simulink model "Geometric_Controller"  (R2021a)
settings: Solver=FixedStepAuto  StartTime=0.0  StopTime=40  FixedStep=0.001  RelTol=1e-3
values from neighbouring files (symbols this model uses):
  g = 9.81    [init.m]
  I = 0.025*eye(3)    [init.m]
  m = 1.5    [init.m]
  omega_0 = [0 0 0]    [init.m]
  p_0 = [0 0 0]    [init.m]
  R_0 = eye(3)    [init.m]
  V_0 = [0 0 0]    [init.m]
libraries: vrlib x2, sharedtransform x1
settings Model: Creator=RyllM  LastModifiedBy=RyllM
settings SolverCC: AlgebraicLoopSolver=TrustRegion
settings DataIOCC: ReturnWorkspaceOutputs=off
settings DebuggingCC: SFMachineParentedDataDiag=warning  ArithmeticOperatorsInVariantConditions=warning
settings SFSimCC: SimUseLocalCustomCode=off  CustomCodeUndefinedFunction=UseInterfaceOnly
settings RTWCC: RTWUseLocalCustomCode=off
settings CodeAppCC: StateflowObjectComments=on

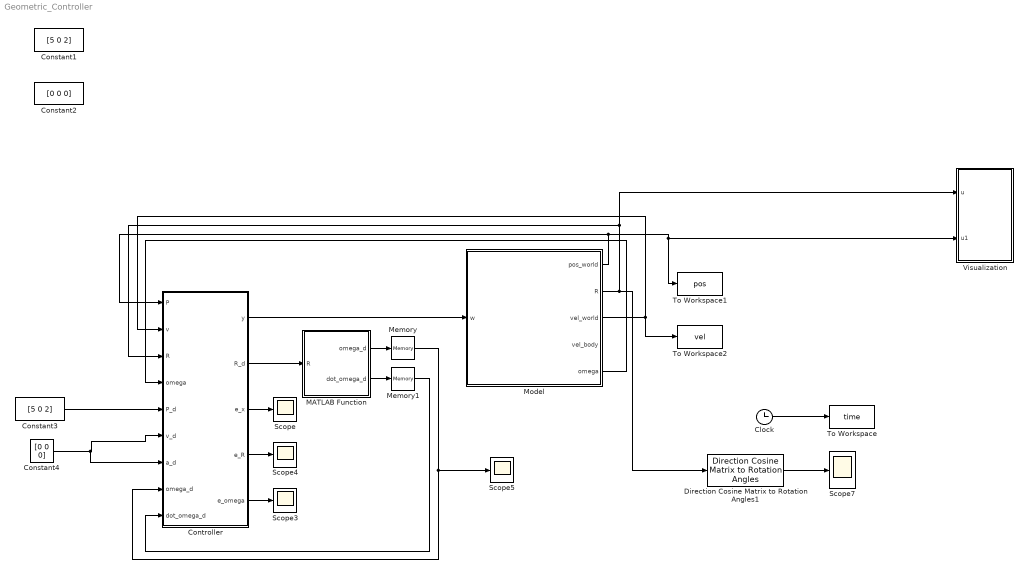
== system Geometric_Controller ==
  Clock : Clock
  Constant1 : Constant  Value=[5 0 2]
  Constant2 : Constant  Value=[0 0 0]
  Constant3 : Constant  Value=[5 0 2]
  Constant4 : Constant  Value=[0 0 0]
  Controller : MATLAB Function  TreatAsAtomicUnit=on
  Direction Cosine Matrix to Rotation Angles1 : sharedtransform/Direction Cosine Matrix to Rotation Angles  rotationOrder=ZYX  aMode=aMode  action=None  tolerance=eps(2)
      settings: SourceProductBaseCode=AE,PW,DR,MT,UV,VE
  MATLAB Function : MATLAB Function  TreatAsAtomicUnit=on
  Memory : Memory  InitialCondition=zeros(3,1)  InheritSampleTime=on
  Memory1 : Memory  InitialCondition=zeros(3,1)  InheritSampleTime=on
  Model : Subsystem
  Scope{,3..5,7} (5 alike) : Scope
  To Workspace : ToWorkspace  VariableName=time  SampleTime=-1
  To Workspace1 : ToWorkspace  VariableName=pos  SampleTime=-1
  To Workspace2 : ToWorkspace  VariableName=vel  SampleTime=-1
  Visualization : Subsystem
  wires:
  Model/1(pos_world) -> Controller/1(P), Visualization/2(u1), To Workspace1/1
  Model/5(omega) -> Controller/4(omega)
  Clock/1 -> To Workspace/1
  Model/3(vel_world) -> Controller/2(v), To Workspace2/1
  Constant4/1 -> Controller/7(a_d), Controller/6(v_d)
  Controller/1(y) -> Model/1(w)
  Controller/3(e_x) -> Scope/1
  Controller/2(R_d) -> MATLAB Function/1(R)
  MATLAB Function/1(omega_d) -> Memory/1
  Memory/1 -> Scope5/1, Controller/8(omega_d)
  Controller/4(e_R) -> Scope4/1
  MATLAB Function/2(dot_omega_d) -> Memory1/1
  Model/2(R) -> Direction Cosine Matrix to Rotation Angles1/1, Visualization/1(u), Controller/3(R)
  Direction Cosine Matrix to Rotation Angles1/1 -> Scope7/1
  Memory1/1 -> Controller/9(dot_omega_d)
  Controller/5(e_omega) -> Scope3/1
  Constant3/1 -> Controller/5(P_d)

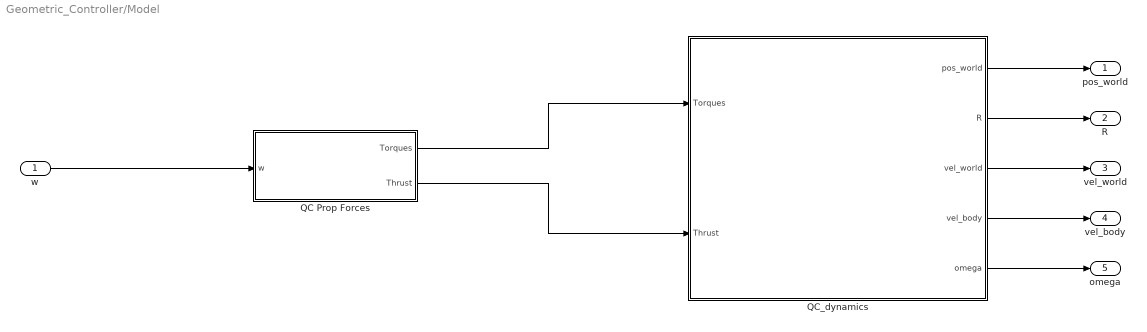
== system Geometric_Controller/Model ==
  w : Inport
  QC Prop Forces : MATLAB Function  TreatAsAtomicUnit=on
  QC_dynamics : Subsystem
  pos_world : Outport
  R : Outport  Port=2
  vel_world : Outport  Port=3
  vel_body : Outport  Port=4
  omega : Outport  Port=5
  wires:
  QC Prop Forces/1(Torques) -> QC_dynamics/1(Torques)
  QC Prop Forces/2(Thrust) -> QC_dynamics/2(Thrust)
  QC_dynamics/1(pos_world) -> pos_world/1
  QC_dynamics/2(R) -> R/1
  QC_dynamics/3(vel_world) -> vel_world/1
  QC_dynamics/4(vel_body) -> vel_body/1
  QC_dynamics/5(omega) -> omega/1
  w/1 -> QC Prop Forces/1(w)

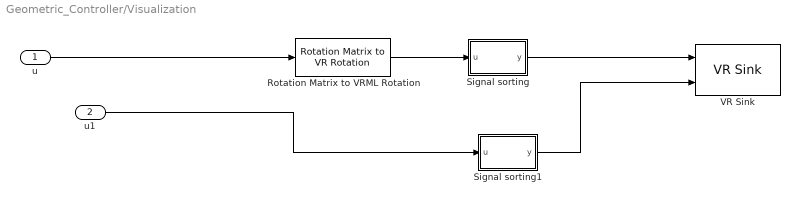
== system Geometric_Controller/Visualization ==
  u : Inport
  u1 : Inport  Port=2
  Rotation Matrix to VRML Rotation : vrlib/Utilities/Rotation Matrix to VR Rotation  maxzero=1e-12
      settings: SourceProductBaseCode=SL
  Signal sorting : MATLAB Function  TreatAsAtomicUnit=on
  Signal sorting1 : MATLAB Function  TreatAsAtomicUnit=on
  VR Sink : vrlib/VR Sink  InstantiateOnLoad=on  SampleTime=0.1  ViewEnable=on  RemoteChange=off  RemoteView=off  FieldsWritten=Quad.rotation.4.1.1.double#Quad.translation.3.1.1.double  WorldFileName=Quad.wrl  AutoView=off  VideoDimensions=[]  AllowVariableSize=off  FigureProperties="{'Position', 'Name', 'Viewpoint', 'CameraBound', 'CameraDirection', 'CameraPosition', 'CameraUpVector', 'ZoomFactor', 'Antialiasing', 'Headlight', 'Lighting', 'NavPanel', 'Sound', 'StatusBar', 'Stereo3D', 'Stereo3DCameraOffset', 'Stereo3DHIT', 'ToolBar', 'Textures', 'Transparency', 'Triad', 'Wireframe', 'NavZones', 'NavMode', 'NavSpeed', 'CaptureFileFormat', 'CaptureFileName', 'Record2DCompressMethod', 'Record2DCompressQuality', 'Record2D', 'Record2DFileName', 'Record2DFPS'; [1.9210000000000000e+03   7.6000000000000000e+01   1.9200000000000000e+03   9.1300000000000000e+02], '', '_untitled_1', 'on', [0.0000000000000000e+00   0.0000000000000000e+00  -1.0000000000000000e+00], [0.0000000000000000e+00   0.0000000000000000e+00   3.0000000000000000e+00], [0.0000000000000000e+00   1.0000000000000000e+00   0.0000000000000000e+00], [1.0000000000000000e+00], 'on', 'on', 'on', 'halfbar', 'on', 'on', 'off', [1.0000000149011612e-01], [0.0000000000000000e+00], 'on', 'on', 'on', 'none', 'off', 'off', 'fly', 'normal', 'tif', '%f_anim_%n.tif', 'auto', [7.5000000000000000e+01], 'off', '%f_anim_%n.avi', 'auto'}"
  wires:
  Rotation Matrix to VRML Rotation/1 -> Signal sorting/1(u)
  u/1 -> Rotation Matrix to VRML Rotation/1
  Signal sorting/1(y) -> VR Sink/1
  Signal sorting1/1(y) -> VR Sink/2
  u1/1 -> Signal sorting1/1(u)

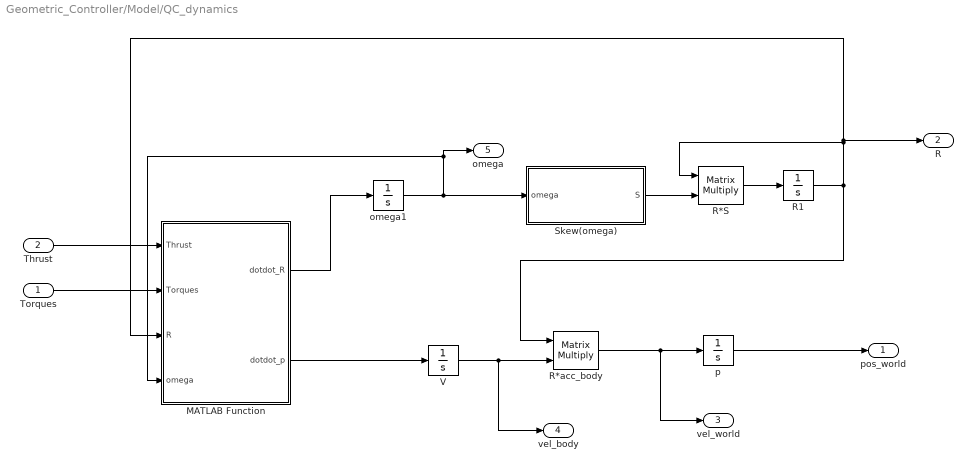
== system Geometric_Controller/Model/QC_dynamics ==
  Torques : Inport
  Thrust : Inport  Port=2
  MATLAB Function : MATLAB Function  TreatAsAtomicUnit=on
  R*S : Product  Multiplication=Matrix(*)  RndMeth=Zero
  R*acc_body : Product  Multiplication=Matrix(*)  RndMeth=Zero
  R1 : Integrator  InitialCondition=R_0
  Skew(omega) : MATLAB Function  TreatAsAtomicUnit=on
  V : Integrator  InitialCondition=V_0
  omega1 : Integrator  InitialCondition=omega_0
  p : Integrator  InitialCondition=p_0
  pos_world : Outport
  R : Outport  Port=2
  vel_world : Outport  Port=3
  vel_body : Outport  Port=4
  omega : Outport  Port=5
  wires:
  V/1 -> R*acc_body/2, vel_body/1
  omega1/1 -> Skew(omega)/1(omega), omega/1, MATLAB Function/4(omega)
  R*S/1 -> R1/1
  R1/1 -> MATLAB Function/3(R), R/1, R*S/1, R*acc_body/1
  Skew(omega)/1(S) -> R*S/2
  Torques/1 -> MATLAB Function/2(Torques)
  p/1 -> pos_world/1
  R*acc_body/1 -> vel_world/1, p/1
  Thrust/1 -> MATLAB Function/1(Thrust)
  MATLAB Function/1(dotdot_R) -> omega1/1
  MATLAB Function/2(dotdot_p) -> V/1

== matlab function Geometric_Controller/Controller ==
  data: P input; y output; R_d output; v input; R input; omega input; P_d input; v_d input; a_d input; omega_d input; dot_omega_d input; m parameter; g parameter; I parameter; e_x output; e_R output; e_omega output
function [y, R_d, e_x, e_R, e_omega] = fcn(P, v, R, omega, P_d, v_d, a_d, omega_d, dot_omega_d, m, g, I)


k_x = 10;
k_v = 8;
k_R = 12;
k_omega = 8;

% dot_omega_d=[0;0;0];


e_x = P_d - P;
e_v = v_d - v;

b1_d = [1;0;0];
%omega_d = [0;0;0];

if(  norm(k_x*e_x + k_v*e_v - m*g*[0;0;-1] + m*a_d) < 0.1)
    b3_d=(k_x*e_x + k_v*e_v - m*g*[0;0;-1] + m*a_d) / 0.1;
else
    b3_d=(k_x*e_x + k_v*e_v - m*g*[0;0;-1] + m*a_d) / norm(k_x*e_x + k_v*e_v - m*g*[0;0;-1] + m*a_d);
end

b2_d = cross(b3_d, b1_d) / norm(cross(b3_d, b1_d));
b1_d = cross(b2_d, b3_d) / norm(cross(b2_d, b3_d));

R_d = [b1_d b2_d b3_d]';


E_R = 1/2 * (R_d'*R - R'*R_d);
e_R = [E_R(3,2); E_R(1,3); E_R(2,1)];
e_omega = omega - R'*R_d*omega_d;
J=I;


omega_h = [0 -omega(3) omega(2);...
           omega(3) 0 -omega(1);...
           -omega(2) omega(1) 0];


f = (k_x*e_x + k_v*e_v + m*g*[0;0;1] + m*a_d)' * R * [0;0;1];
M = -k_R*e_R - k_omega * e_omega+cross(omega,J*omega)-J*(omega_h*R'*R_d*omega_d-R'*R_d*dot_omega_d);

y = [f; M];

== matlab function Geometric_Controller/Model/QC Prop Forces ==
  data: w input; Torques output; Thrust output; T_act parameter
function [Torques, Thrust]= fcn(w, T_act)
% This block supports the Embedded MATLAB subset.
% See the help menu for details. 


Thrust=[0;0;w(1)];

Torques=w(2:4);

== matlab function Geometric_Controller/Visualization/Signal sorting ==
  data: u input; y output
function y = fcn(u)

y = [u(2) u(2) u(2) u(4)];

== matlab function Geometric_Controller/Visualization/Signal sorting1 ==
  data: u input; y output
function y = fcn(u)

y = [u(1) u(3) -u(2)];

== matlab function Geometric_Controller/MATLAB Function ==
  settings: updateMethod=DISCRETE
  data: R input; omega_d output; basic_time_step parameter; dot_omega_d output
function [omega_d, dot_omega_d] = fcn(R, basic_time_step)

persistent R_previous;
persistent omega_d_previous;

if isempty(R_previous)
    R_previous = eye(3);
end

if isempty(omega_d_previous)
    omega_d_previous = zeros(3,1);
end
    

R_dot = (R - R_previous)/basic_time_step;

omega_d_skew = (R_dot * R');

omega_d = [omega_d_skew(3,2) omega_d_skew(1,3) omega_d_skew(2,1)]';
dot_omega_d = (omega_d - omega_d_previous)/basic_time_step;

if norm(omega_d)>100
    omega_d = [0;0;0];
end

if norm(dot_omega_d)>50
    dot_omega_d = [0;0;0];
end

R_previous = R;
omega_d_previous = omega_d;

== matlab function Geometric_Controller/Model/QC_dynamics/MATLAB Function ==
  data: dotdot_R output; Thrust input; dotdot_p output; Torques input; R input; omega input; m parameter; g parameter; I parameter
function [dotdot_R, dotdot_p] = fcn(Thrust, Torques, R, omega, m, g, I)

dotdot_p = (Thrust / m - R*[0; 0; g]);

dotdot_R = I^-1*(Torques - cross(omega, I * omega));

== matlab function Geometric_Controller/Model/QC_dynamics/Skew(omega) ==
  data: omega input; S output
function S = skew(omega)
% This block supports the Embedded MATLAB subset.
% See the help menu for details. 
S = [0 -omega(3) omega(2);
 omega(3) 0 -omega(1);
 -omega(2) omega(1) 0];
